simulink model "z_1.1"  (R2022b)
settings: Solver=VariableStepAuto  StartTime=0.0  StopTime=10.0  RelTol=1e-3
libraries: simulink x3
settings Model: Creator=amirz  LastModifiedBy=amirz

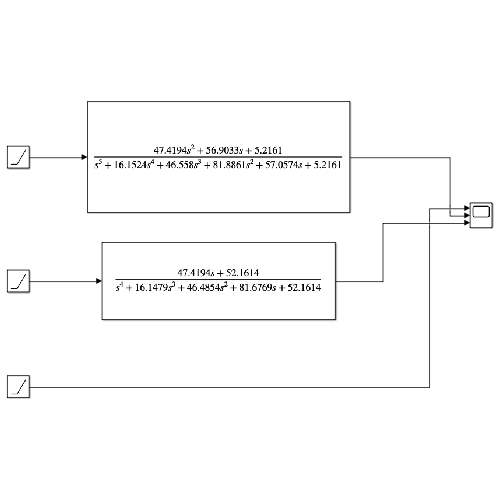
[thumbnail: Simulink's stored preview of the top-level diagram]
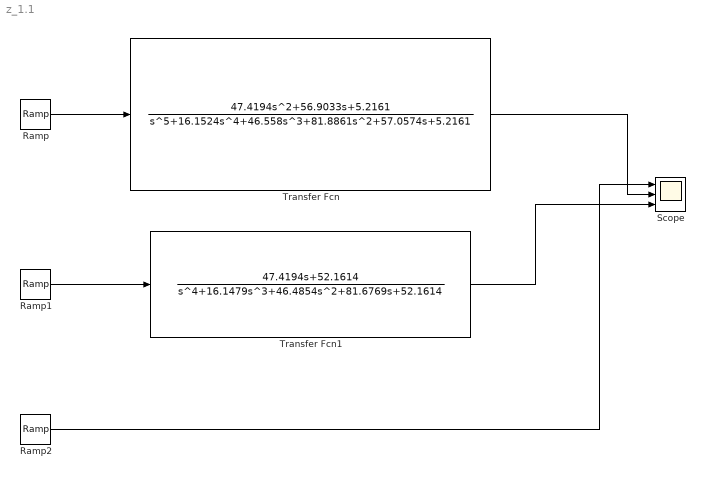
== system z_1.1 ==
  Ramp : simulink/Sources/Ramp  slope=1  start=0  InitialOutput=0
  Ramp1 : simulink/Sources/Ramp  slope=1  start=0  InitialOutput=0
  Ramp2 : simulink/Sources/Ramp  slope=1  start=0  InitialOutput=0
  Scope : Scope  NumInputPorts=3
  Transfer Fcn : TransferFcn  Numerator=[47.4194 56.9033 5.2161]  Denominator=[1 16.1524 46.558 81.8861 57.0574 5.2161]
  Transfer Fcn1 : TransferFcn  Numerator=[47.4194 52.1614]  Denominator=[1 16.1479 46.4854 81.6769 52.1614]
  wires:
  Ramp/1 -> Transfer Fcn/1
  Ramp1/1 -> Transfer Fcn1/1
  Ramp2/1 -> Scope/1
  Transfer Fcn1/1 -> Scope/3
  Transfer Fcn/1 -> Scope/2
